simulink model "kalman_filter_sim"  (R2016a)
settings: Solver=VariableStepAuto  StartTime=0.0  StopTime=10.0  RelTol=1e-3
undefined symbols (not defined in the file or in its folder): Discete_Kalman_filter
settings Model: Creator=zhanghankui  LastModifiedBy=zhanghankui

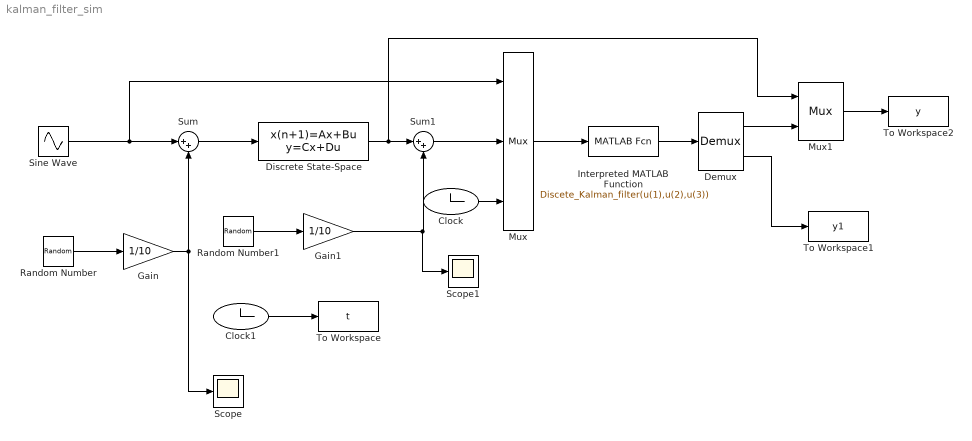
== system kalman_filter_sim ==
  Clock : Clock
  Clock1 : Clock
  Demux : Demux  Outputs=2
  Discrete State-Space : DiscreteStateSpace  A=[1.0000 0.0010;0 0.9753]  B=[0.0001;0.1314]  C=[1 0]  D=0  SampleTime=0.001
  Gain : Gain  Gain=1/10
  Gain1 : Gain  Gain=1/10
  Interpreted MATLAB Function : MATLABFcn  MATLABFcn=Discete_Kalman_filter(u(1),u(2),u(3))  OutputDimensions=2
  Mux : Mux  Inputs=3
  Mux1 : Mux  Inputs=2
  Random Number : RandomNumber  SampleTime=0.1
  Random Number1 : RandomNumber  SampleTime=0.1
  Scope : Scope
  Scope1 : Scope
  Sine Wave : Sin  Frequency=0.5*2*pi  SampleTime=0
  Sum : Sum  Inputs=|++
  Sum1 : Sum  Inputs=|++
  To Workspace : ToWorkspace  VariableName=t  SampleTime=-1
  To Workspace1 : ToWorkspace  VariableName=y1  SampleTime=-1
  To Workspace2 : ToWorkspace  VariableName=y  SampleTime=-1
  wires:
  Random Number/1 -> Gain/1
  Sine Wave/1 -> Mux/1, Sum/1
  Gain/1 -> Scope/1, Sum/2
  Sum/1 -> Discrete State-Space/1
  Random Number1/1 -> Gain1/1
  Discrete State-Space/1 -> Mux1/1, Sum1/1
  Gain1/1 -> Scope1/1, Sum1/2
  Sum1/1 -> Mux/2
  Clock/1 -> Mux/3
  Mux/1 -> Interpreted MATLAB Function/1
  Clock1/1 -> To Workspace/1
  Interpreted MATLAB Function/1 -> Demux/1
  Demux/2 -> To Workspace1/1
  Demux/1 -> Mux1/2
  Mux1/1 -> To Workspace2/1
